simulink model "OutputToStimulatorOnNextTrigger"  (R2016b)
settings: Solver=FixedStepDiscrete  StartTime=0.0  StopTime=inf  FixedStep=sCoreParams.core.stepPeriod  RelTol=1e-3
undefined symbols (not defined in the file): Low, sCoreParams, sCoreParams_stimulator_refractoryPeriodSec, sCoreParams_stimulator_startupTimeSec
libraries: dspswit3 x3, simulink x2, xpcparallelportlib x1
Description:
  | This model consists of the simulator configuration and the output to the parallel port.
  | Inputs:
  |   1. isEventDetected: 1 if event was detected 0 if NO event.
  |   2. sendStimPulse: 1 if a stimulus should be sent
  | An example of the usage if this two inputs follows. We could have 2 reason to perform a stimulation (e.g. event detected or sham).
  | In that case input 1 will be 1 only when event is detected while input 2 will be 1 for both stimulations.
  | 
  | Outputs:
  |   1. StimHappening: Indicates that a stimulation pulse was sent through the parallel port to the cerexstim
settings Model: DataTypeOverride=Double  MinMaxOverflowLogging=ForceOff  Creator=rzelmann  LastModifiedBy=rzelmann
settings SolverCC: EnableConcurrentExecution=on  AutoInsertRateTranBlk=on
settings DataIOCC: LimitDataPoints=on  SaveFormat=StructureWithTime  SaveOutput=off  SignalLogging=off  SaveTime=off
settings OptimizationCC: BlockReduction=off  DefaultParameterBehavior=Inlined  OptimizeBlockIOStorage=off  BufferReuse=off  GlobalBufferReuse=off  ExpressionFolding=off  LocalBlockOutputs=off  LifeSpan=inf
settings DebuggingCC: AlgebraicLoopMsg=error  SingleTaskRateTransMsg=error  AllowSymbolicDim=off  SFUnexpectedBacktrackingDiag=warning  SFNoUnconditionalDefaultTransitionDiag=warning  SFExecutionAtInitializationDiag=none
settings HardwareCC: ProdBitPerPointer=32  ProdBitPerSizeT=32  ProdBitPerPtrDiffT=32  ProdLargestAtomicFloat=None  ProdWordSize=32  ProdLongLongMode=on  ProdHWDeviceType=Generic->32-bit x86 compatible
settings ModelReferenceCC: ModelReferenceNumInstancesAllowed=Single  ModelReferencePassRootInputsByReference=off
settings RTWCC: SystemTargetFile=slrt.tlc  TemplateMakefile=slrt_default_tmf  Description=Simulink Real-Time  RTWCompilerOptimization=on
settings ConfigComp: CovMetricSettings=dw  CovHtmlReporting=on  CovSaveCumulativeToWorkspaceVar=on  CovSaveSingleToWorkspaceVar=on  CovExternalEMLEnable=off

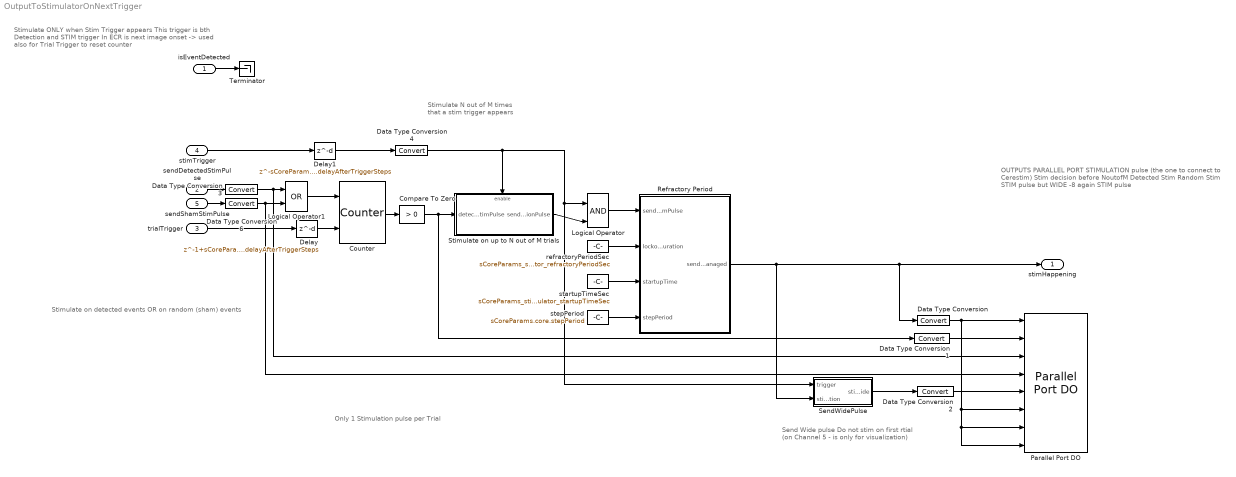
== system OutputToStimulatorOnNextTrigger ==
  note: Send Wide pulse
      | Do not stim on first rtial
      | (on Channel 5 - is only for visualization)
  note: Only 1 Stimulation pulse per Trial
  note: Stimulate N out of M times
      | that a stim trigger appears
  note: OUTPUTS PARALLEL PORT
      | STIMULATION pulse (the one to connect to Cerestim)
      | Stim decision before NoutofM
      | Detected Stim
      | Random Stim
      | STIM pulse but WIDE
      | -8 again STIM pulse
  note: Stimulate on detected events OR on random (sham) events
  note: Stimulate ONLY when Stim Trigger appears
      | This trigger is bth Detection and STIM trigger
      | In ECR is next image onset -> used also for Trial Trigger to
      | reset counter
  isEventDetected : Inport  OutDataTypeStr=boolean  SampleTime=sCoreParams.core.stepPeriod
  sendDetectedStimPulse : Inport  Port=2  OutDataTypeStr=boolean  SampleTime=sCoreParams.core.stepPeriod
  trialTrigger : Inport  Port=3  OutDataTypeStr=int32  SampleTime=sCoreParams.core.stepPeriod
  stimTrigger : Inport  Port=4  OutDataTypeStr=int32  SampleTime=sCoreParams.core.stepPeriod
  sendShamStimPulse : Inport  Port=5  OutDataTypeStr=boolean  SampleTime=sCoreParams.core.stepPeriod
  Compare To Zero : simulink/Logic and Bit Operations/Compare To Zero  relop=>  OutDataTypeStr=boolean
  Counter : dspswit3/Counter  Direction=Up  CountEvent=Non-zero sample  CounterSize=16 bits  MaxCount=sCoreParams.decoders.txDetector.detectionDurationSamples  InitialCount=0  Output=Count  HitValue=sCoreParams.decoders.txDetector.detectionDurationSamples  ResetInput=on  SamplesPerFrame=1  Ts=sCoreParams.core.stepPeriod  CntDtype=int32  HitDtype=Logical
  Data Type Conversion{,1..4,6} (6 alike) : DataTypeConversion
  Delay : Delay  DelayLength=1+sCoreParams.stimulator.delayAfterTriggerSteps
  Delay1 : Delay  DelayLength=sCoreParams.stimulator.delayAfterTriggerSteps
  Logical Operator : Logic  IconShape=distinctive  AllPortsSameDT=off  OutDataTypeStr=boolean
  Logical Operator1 : Logic  Operator=OR  IconShape=distinctive  AllPortsSameDT=off  OutDataTypeStr=boolean
  "Parallel Port DO " : xpcparallelportlib/Digital Output/Parallel Port DO   BaseMask=0x378  BaseString=0x378  Format=8 1-bit Channels  Channels=[1:8]  InitialValues=[0]  FinalActions=[0]  FinalValues=[0]  SampleTime=sCoreParams.core.stepPeriod  Mode=1
  Refractory Period : MATLAB Function  TreatAsAtomicUnit=on  SystemSampleTime=sCoreParams.core.stepPeriod
  SendWidePulse : Subsystem
  Stimulate on up to N out of M trials : Subsystem
  Terminator : Terminator
  refractoryPeriodSec : Constant  Value=sCoreParams_stimulator_refractoryPeriodSec
  startupTimeSec : Constant  Value=sCoreParams_stimulator_startupTimeSec
  stepPeriod : Constant  Value=sCoreParams.core.stepPeriod
  stimHappening : Outport  OutDataTypeStr=boolean  SampleTime=sCoreParams.core.stepPeriod
  wires:
  stepPeriod/1 -> Refractory Period/4(stepPeriod)
  startupTimeSec/1 -> Refractory Period/3(startupTime)
  refractoryPeriodSec/1 -> Refractory Period/2(lockoutDuration)
  Data Type Conversion/1 -> "Parallel Port DO "/8, "Parallel Port DO "/7, "Parallel Port DO "/6, "Parallel Port DO "/1
  Counter/1 -> Compare To Zero/1
  trialTrigger/1 -> Delay/1
  stimTrigger/1 -> Delay1/1
  Compare To Zero/1 -> Data Type Conversion1/1, Stimulate on up to N out of M trials/1(detectedStimPulse)
  Logical Operator/1 -> Refractory Period/1(sendStimPulse)
  Logical Operator1/1 -> Counter/1
  Delay/1 -> Counter/2
  Delay1/1 -> Data Type Conversion4/1
  sendDetectedStimPulse/1 -> Data Type Conversion3/1
  sendShamStimPulse/1 -> Data Type Conversion6/1
  Data Type Conversion3/1 -> "Parallel Port DO "/3, Logical Operator1/1
  Data Type Conversion6/1 -> "Parallel Port DO "/4, Logical Operator1/2
  Data Type Conversion1/1 -> "Parallel Port DO "/2
  isEventDetected/1 -> Terminator/1
  Data Type Conversion4/1 -> Stimulate on up to N out of M trials/Enable, SendWidePulse/1(trigger), Logical Operator/1
  Stimulate on up to N out of M trials/1(sendStimulationPulse) -> Logical Operator/2
  Refractory Period/1(sendStimManaged) -> SendWidePulse/2(stimulation), stimHappening/1, Data Type Conversion/1
  SendWidePulse/1(stimulationWide) -> Data Type Conversion2/1
  Data Type Conversion2/1 -> "Parallel Port DO "/5

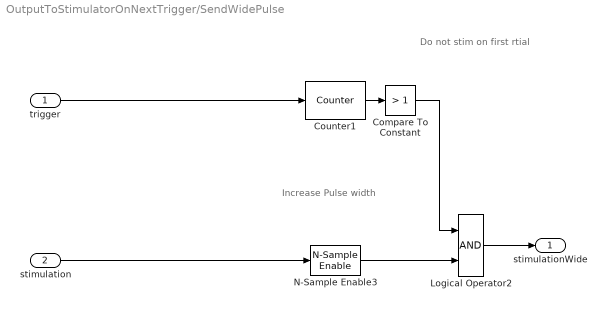
== system OutputToStimulatorOnNextTrigger/SendWidePulse ==
  note: Increase Pulse width
  note: Do not stim on first rtial
  trigger : Inport
  stimulation : Inport  Port=2
  Compare To Constant : simulink/Logic and Bit Operations/Compare To Constant  relop=>  const=1  OutDataTypeStr=boolean
  Counter1 : dspswit3/Counter  Direction=Up  CountEvent=Rising edge  CounterSize=16 bits  MaxCount=sCoreParams.decoders.txDetector.detectionDurationSamples  InitialCount=0  Output=Count  HitValue=sCoreParams.decoders.txDetector.detectionDurationSamples  ResetInput=off  SamplesPerFrame=1  Ts=sCoreParams.core.stepPeriod  CntDtype=int32  HitDtype=Logical
  Logical Operator2 : Logic  IconShape=distinctive  AllPortsSameDT=off  OutDataTypeStr=boolean
  N-Sample Enable3 : dspswit3/N-Sample Enable  N=sCoreParams.viz.pulseWidthStimSteps  ActiveLevel=Low (0)  reset=on  TriggerType=Rising edge  Ts=1  DataType=Logical
  stimulationWide : Outport
  wires:
  N-Sample Enable3/1 -> Logical Operator2/2
  Logical Operator2/1 -> stimulationWide/1
  stimulation/1 -> N-Sample Enable3/1
  Counter1/1 -> Compare To Constant/1
  Compare To Constant/1 -> Logical Operator2/1
  trigger/1 -> Counter1/1

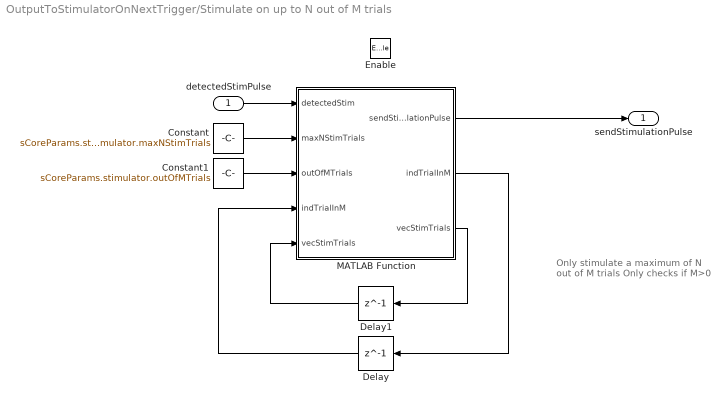
== system OutputToStimulatorOnNextTrigger/Stimulate on up to N out of M trials ==
  note: Only stimulate a maximum of N
      |  out of M trials
      | Only checks if M>0
  detectedStimPulse : Inport  OutDataTypeStr=boolean
  Enable : EnablePort
  Constant : Constant  Value=sCoreParams.stimulator.maxNStimTrials
  Constant1 : Constant  Value=sCoreParams.stimulator.outOfMTrials
  Delay : Delay  DelayLength=1  InitialCondition=0
  Delay1 : Delay  DelayLength=1  InitialCondition=zeros(sCoreParams.stimulator.outOfMTrials,1)
  MATLAB Function : MATLAB Function  TreatAsAtomicUnit=on
  sendStimulationPulse : Outport  OutputWhenDisabled=reset  InitialOutput=0
  wires:
  MATLAB Function/1(sendStimulationPulse) -> sendStimulationPulse/1
  detectedStimPulse/1 -> MATLAB Function/1(detectedStim)
  Constant/1 -> MATLAB Function/2(maxNStimTrials)
  Constant1/1 -> MATLAB Function/3(outOfMTrials)
  MATLAB Function/2(indTrialInM) -> Delay/1
  Delay/1 -> MATLAB Function/4("indTrialInM ")
  MATLAB Function/3(vecStimTrials) -> Delay1/1
  Delay1/1 -> MATLAB Function/5("vecStimTrials ")

== matlab function OutputToStimulatorOnNextTrigger/Stimulate on up to N out of M trials/MATLAB Function ==
  data: detectedStim input; sendStimulationPulse output; maxNStimTrials input; outOfMTrials input; indTrialInM input; vecStimTrials input; indTrialInM output; vecStimTrials output
function [sendStimulationPulse, indTrialInM, vecStimTrials]  = fcnStimulateNoutofMtrials(detectedStim, maxNStimTrials, outOfMTrials,  indTrialInM, vecStimTrials)

if outOfMTrials>0
    [sendStimulationPulse, indTrialInM, vecStimTrials] = stimulateNoutofMtrials(detectedStim, maxNStimTrials, outOfMTrials, indTrialInM, vecStimTrials);
else
    sendStimulationPulse = detectedStim;
end

== matlab function OutputToStimulatorOnNextTrigger/Refractory Period ==
  data: sendStimPulse input; sendStimManaged output; lockoutDuration input; startupTime input; stepPeriod input
function sendStimManaged = ManageStimLockoutWithProbaStim(sendStimPulse,lockoutDuration,startupTime,stepPeriod)
%#codegen

%sendStimManagedB = ManageStimLockoutWithProbaStim_EML(sendStimPulse,lockoutDuration,startupTime,stepPeriod, probabilityOfStim);
sendStimManaged = ManageStimLockout_EML(sendStimPulse,lockoutDuration,startupTime,stepPeriod);
%sendStimManaged = double(sendStimManagedB);
